simulink model "runSfun2"  (R2019b)
settings: Solver=FixedStepDiscrete  StartTime=340.0  StopTime=350.0  FixedStep=Ts  RelTol=1e-3  EnableMultiTasking=on
settings Model: PauseTimes=341.0  Creator=btc2abt  LastModifiedBy=IGG2BP
settings DataIOCC: LimitDataPoints=on  ReturnWorkspaceOutputs=off
settings OptimizationCC: LifeSpan=inf
settings DebuggingCC: MultiTaskRateTransMsg=warning  AllowSymbolicDim=off  SFUnexpectedBacktrackingDiag=warning  SFNoUnconditionalDefaultTransitionDiag=warning  SFExecutionAtInitializationDiag=none  ArithmeticOperatorsInVariantConditions=warning
settings ModelReferenceCC: PropagateSignalLabelsOutOfModel=off
settings SFSimCC: SimUseLocalCustomCode=off  CustomCodeUndefinedFunction=UseInterfaceOnly
settings RTWCC: RTWUseLocalCustomCode=off
settings CodeAppCC: StateflowObjectComments=on
settings GRTTargetCC: TargetLangStandard=C89/C90 (ANSI)
settings ConfigComp: CovMetricSettings=dw  CovHtmlReporting=on  CovSaveCumulativeToWorkspaceVar=on  CovSaveSingleToWorkspaceVar=on  CovExternalEMLEnable=off

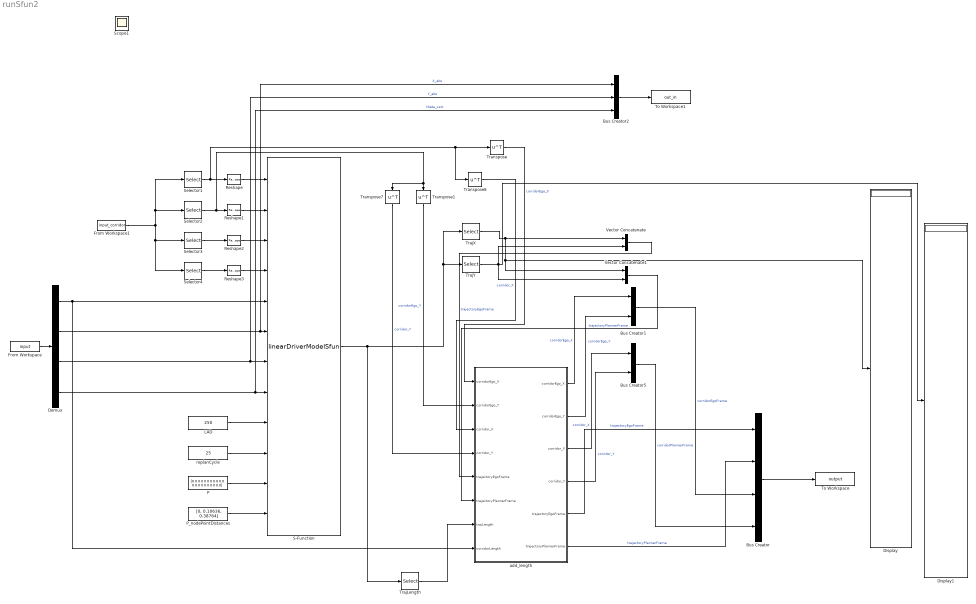
== system runSfun2 ==
  Bus Creator : BusCreator  Inputs=4
  Bus Creator1 : BusCreator  Inputs=2
  Bus Creator2 : BusCreator  Inputs=3
  Bus Creator5 : BusCreator  Inputs=2
  Demux : Demux
  Display : Display
  Display1 : Display
  From Workspace : FromWorkspace  VariableName=input  SampleTime=0  Interpolate=off  OutputAfterFinalValue=Holding final value
  From Workspace1 : FromWorkspace  VariableName=input_corridor  SampleTime=0  Interpolate=off  OutputAfterFinalValue=Holding final value
  LAD : Constant  Value=250
  P : Constant  Value=[0 0 0 0 0 0 0 0 0 0 0 0 0 0 0 0 0 0 0 0 0]
  P_nodePointDistances : Constant  Value=[0, 0.10636, 0.38764]
  Reshape{,1..3} (4 alike) : Reshape
  S-Function : S-Function  FunctionName=linearDriverModelSfun  SFunctionDeploymentMode=off  EnableBusSupport=off
  Selector1 : Selector  NumberOfDimensions=2  InputPortWidth=3  IndexOptions=Index vector (dialog),Select all  Indices=[1],1  OutputSizes=1,1
  Selector2 : Selector  NumberOfDimensions=2  InputPortWidth=3  IndexOptions=Index vector (dialog),Select all  Indices=[2],1  OutputSizes=1,1
  Selector3 : Selector  NumberOfDimensions=2  InputPortWidth=3  IndexOptions=Index vector (dialog),Select all  Indices=[3],1  OutputSizes=1,1
  Selector4 : Selector  NumberOfDimensions=2  InputPortWidth=3  IndexOptions=Index vector (dialog),Select all  Indices=[4],1  OutputSizes=1,1
  To Workspace : ToWorkspace  VariableName=output  SaveFormat=Timeseries  SampleTime=-1
  To Workspace1 : ToWorkspace  VariableName=out_in  SaveFormat=Timeseries  SampleTime=-1
  TrajLength : Selector  InputPortWidth=601  IndexOptions=Index vector (dialog)  Indices=601  OutputSizes=1
  TrajX : Selector  InputPortWidth=601  IndexOptions=Index vector (dialog)  Indices=linspace(1,300,300)  OutputSizes=1
  TrajY : Selector  InputPortWidth=601  IndexOptions=Index vector (dialog)  Indices=linspace(301,600,300)  OutputSizes=1
  Transpose{,1,7..8} (4 alike) : Math  Operator=transpose  SignedPower=off  SaturateOnIntegerOverflow=on
  Vector Concatenate : Concatenate  Mode=Multidimensional array  ConcatenateDimension=2
  Vector Concatenate1 : Concatenate  Mode=Multidimensional array  ConcatenateDimension=2
  add_length : MATLAB Function  TreatAsAtomicUnit=on
  replanCycle : Constant  Value=25
  Scope1 : Scope
  wires:
  P/1 -> S-Function/11
  P_nodePointDistances/1 -> S-Function/12
  replanCycle/1 -> S-Function/10
  LAD/1 -> S-Function/9
  S-Function/1 -> TrajX/1, TrajY/1, TrajLength/1
  From Workspace/1 -> Demux/1
  From Workspace1/1 -> Selector1/1, Selector2/1, Selector3/1, Selector4/1
  Selector1/1 -> Transpose/1, Transpose8/1, Reshape/1
  Selector2/1 -> Transpose7/1, Transpose1/1, Reshape1/1
  Selector3/1 -> Reshape2/1
  Selector4/1 -> Reshape3/1
  Demux/1 -> add_length/8(corridorLength), S-Function/5
  Demux/2 -> Bus Creator2/1, S-Function/6  "X_abs"
  Demux/3 -> S-Function/7, Bus Creator2/2  "Y_abs"
  Demux/4 -> S-Function/8, Bus Creator2/3  "theta_calc"
  Reshape/1 -> S-Function/1
  Reshape1/1 -> S-Function/2
  Reshape2/1 -> S-Function/3
  Reshape3/1 -> S-Function/4
  Bus Creator/1 -> To Workspace/1
  TrajLength/1 -> add_length/7(trajLength)
  Vector Concatenate/1 -> add_length/5("trajectoryEgoFrame ")  "trajectoryEgoFrame"
  TrajX/1 -> Vector Concatenate1/1, Display/1, Vector Concatenate/1
  TrajY/1 -> Vector Concatenate1/2, Vector Concatenate/2, Display1/1
  Transpose/1 -> add_length/1("corridorEgo_X ")  "corridorEgo_X"
  Transpose1/1 -> add_length/2("corridorEgo_Y ")  "corridorEgo_Y"
  Bus Creator2/1 -> To Workspace1/1
  Bus Creator5/1 -> Bus Creator/4  "corridorPlannerFrame"
  Bus Creator1/1 -> Bus Creator/3  "corridorEgoFrame"
  Vector Concatenate1/1 -> add_length/6("trajectoryPlannerFrame ")  "trajectoryPlannerFrame"
  Transpose7/1 -> add_length/4("corridor_Y ")  "corridor_Y"
  Transpose8/1 -> add_length/3("corridor_X ")  "corridor_X"
  add_length/1(corridorEgo_X) -> Bus Creator1/1  "corridorEgo_X"
  add_length/2(corridorEgo_Y) -> Bus Creator1/2  "corridorEgo_Y"
  add_length/3(corridor_X) -> Bus Creator5/1  "corridor_X"
  add_length/4(corridor_Y) -> Bus Creator5/2  "corridor_Y"
  add_length/5(trajectoryEgoFrame) -> Bus Creator/1  "trajectoryEgoFrame"
  add_length/6(trajectoryPlannerFrame) -> Bus Creator/2  "trajectoryPlannerFrame"

== matlab function runSfun2/add_length ==
  data: corridorEgo_X output; corridorEgo_Y output; corridor_X output; corridor_Y output; trajectoryEgoFrame output; trajectoryPlannerFrame output; corridorEgo_X input; corridorEgo_Y input; corridor_X input; corridor_Y input; trajectoryEgoFrame input; trajectoryPlannerFrame input; trajLength input; corridorLength input
function [corridorEgo_X, corridorEgo_Y, corridor_X, corridor_Y, trajectoryEgoFrame, trajectoryPlannerFrame] = add_length(corridorEgo_X, corridorEgo_Y, corridor_X, corridor_Y, trajectoryEgoFrame, trajectoryPlannerFrame, trajLength, corridorLength)

corridorEgo_X(300) = corridorLength;
corridorEgo_Y(300) = corridorLength;
corridor_X(300) = corridorLength;
corridor_Y(300) = corridorLength;
trajectoryEgoFrame(300,:) = trajLength;
trajectoryPlannerFrame(300,:) = trajLength;

end
